simulink model "circuit1"  (R2018a)
settings: Solver=ode5  StartTime=0.0  StopTime=1.0  RelTol=1e-3
libraries: powerlib x24
settings Model: Creator=hanan  LastModifiedBy=hanan

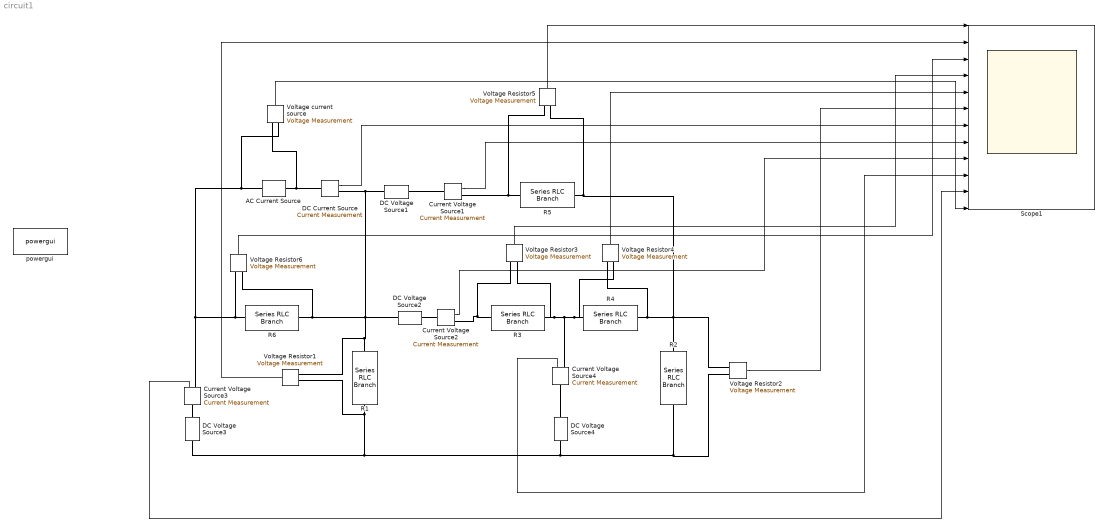
== system circuit1 ==
  " DC Current Source   " : powerlib/Measurements/Current Measurement  PhasorSimulation=off  OutputType=Complex  PSBequivalent=0
  " R1" : powerlib/Elements/Series RLC Branch  LConnTagsString=__new0  RConnTagsString=__new0  BranchType=R  Resistance=1  Inductance=1e-3  SetiL0=off  InitialCurrent=0  Capacitance=1e-6  Setx0=off  InitialVoltage=0  Measurements=Branch voltage
  " R2" : powerlib/Elements/Series RLC Branch  LConnTagsString=__new0  RConnTagsString=__new0  BranchType=R  Resistance=1  Inductance=1e-3  SetiL0=off  InitialCurrent=0  Capacitance=1e-6  Setx0=off  InitialVoltage=0  Measurements=None
  " R3" : powerlib/Elements/Series RLC Branch  LConnTagsString=__new0  RConnTagsString=__new0  BranchType=R  Resistance=1  Inductance=1e-3  SetiL0=off  InitialCurrent=0  Capacitance=1e-6  Setx0=off  InitialVoltage=0  Measurements=None
  " R4" : powerlib/Elements/Series RLC Branch  LConnTagsString=__new0  RConnTagsString=__new0  BranchType=R  Resistance=0.25  Inductance=1e-3  SetiL0=off  InitialCurrent=0  Capacitance=1e-6  Setx0=off  InitialVoltage=0  Measurements=None
  " R5" : powerlib/Elements/Series RLC Branch  LConnTagsString=__new0  RConnTagsString=__new0  BranchType=R  Resistance=0.25  Inductance=1e-3  SetiL0=off  InitialCurrent=0  Capacitance=1e-6  Setx0=off  InitialVoltage=0  Measurements=None
  " R6" : powerlib/Elements/Series RLC Branch  LConnTagsString=__new0  RConnTagsString=__new0  BranchType=R  Resistance=0.5  Inductance=1e-3  SetiL0=off  InitialCurrent=0  Capacitance=1e-6  Setx0=off  InitialVoltage=0  Measurements=None
  AC Current Source : powerlib/Electrical Sources/AC Current Source  Amplitude=2  Phase=90  Frequency=0  SampleTime=0  Measurements=Current
      settings: SourceProductName=Simscape Power Systems  SourceProductBaseCode=PS
  Current Voltage Source{1..4} (4 alike) : powerlib/Measurements/Current Measurement  PhasorSimulation=off  OutputType=Complex  PSBequivalent=0
  DC Voltage Source1 : powerlib/Electrical Sources/DC Voltage Source  Amplitude=2  Measurements=None
  DC Voltage Source2 : powerlib/Electrical Sources/DC Voltage Source  Amplitude=3  Measurements=None
  DC Voltage Source3 : powerlib/Electrical Sources/DC Voltage Source  Amplitude=2  Measurements=None
  DC Voltage Source4 : powerlib/Electrical Sources/DC Voltage Source  Amplitude=0.2977  Measurements=None
  Scope1 : Scope  NumInputPorts=12
  Voltage Resistor{1..6} (6 alike) : powerlib/Measurements/Voltage Measurement  PhasorSimulation=off  OutputType=Complex  PSBequivalent=0
  Voltage current source : powerlib/Measurements/Voltage Measurement  PhasorSimulation=off  OutputType=Complex  PSBequivalent=0
  powergui : powerlib/powergui  Priority=1  SimulationMode=Discrete  SampleTime=50e-6  frequency=60  Iterations=50  frequencyindice=0  Pbase=100e6  ErrMax=1e-4  UnitsV=kV  UnitsW=MW  buscounter=0  FunctionMessages=off  echomessages=off  EnableUseOfTLC=off  CurrentSourceSwitches=off  DisableSnubberDevices=off  DisableRonSwitches=off  DisableVfSwitches=off  DisplayEquations=off  SolverType=Tustin/Backward Euler (TBE)  Interpol=off  ExternalGateDelay=off  methode=off  Ts=100  x0status=blocks  SPID=on  SwTol=0  HookPort=off  RestoreLinks=warning  ResistiveCurrentMeasurement=off  Frange=[0:2:500]  Ylog=off  Xlog=on  ShowGrid=off  save=off  variable=ZData  structure=0  ZoomFFT=off  StartTime=0.0  cycles=1  DisplayStyle=1  fundamental=60  FreqAxis=off  MaxFrequency=1000  frequencyindicesteady=1  RmsSteady=1  display=off
  wires:
  Voltage Resistor5/1 -> Scope1/1
  Voltage Resistor4/1 -> Scope1/5
  Voltage Resistor3/1 -> Scope1/4
  Voltage Resistor6/1 -> Scope1/3
  Voltage Resistor1/1 -> Scope1/2
  Voltage Resistor2/1 -> Scope1/6
  " DC Current Source   "/1 -> Scope1/7
  Current Voltage Source3/1 -> Scope1/11
  Current Voltage Source4/1 -> Scope1/10
  Current Voltage Source1/1 -> Scope1/8
  Current Voltage Source2/1 -> Scope1/9
  Voltage current source/1 -> Scope1/12
  connections:
  " R5"/LConn1 -- Current Voltage Source1/RConn1 -- Voltage Resistor5/LConn1
  Voltage Resistor4/LConn1 -- " R4"/LConn1 -- " R2"/LConn1 -- Voltage Resistor2/LConn1 -- Voltage Resistor5/LConn2 -- " R5"/RConn1
  " R3"/RConn1 -- Voltage Resistor3/LConn2 -- Current Voltage Source4/RConn1 -- Voltage Resistor4/LConn2 -- " R4"/RConn1
  DC Voltage Source3/LConn1 -- Voltage Resistor1/LConn1 -- " R1"/LConn1 -- DC Voltage Source4/LConn1 -- Voltage Resistor2/LConn2 -- " R2"/RConn1
  Voltage Resistor1/LConn2 -- " R1"/RConn1 -- DC Voltage Source2/LConn1 -- DC Voltage Source1/LConn1 -- " DC Current Source   "/RConn1 -- " R6"/RConn1 -- Voltage Resistor6/LConn2
  Voltage Resistor3/LConn1 -- Current Voltage Source2/RConn1 -- " R3"/LConn1
  AC Current Source/LConn1 -- Voltage current source/LConn2 -- " R6"/LConn1 -- Voltage Resistor6/LConn1 -- Current Voltage Source3/RConn1
  AC Current Source/RConn1 -- Voltage current source/LConn1 -- " DC Current Source   "/LConn1
  Current Voltage Source4/LConn1 -- DC Voltage Source4/RConn1
  Current Voltage Source3/LConn1 -- DC Voltage Source3/RConn1
  Current Voltage Source2/LConn1 -- DC Voltage Source2/RConn1
  Current Voltage Source1/LConn1 -- DC Voltage Source1/RConn1
